simulink model "truckaso2"  (R2022b)
settings: Solver=ode3  StartTime=0.0  StopTime=Timesim  FixedStep=0.1  MaxStep=0.1  RelTol=1e-3  AbsTol=1e-6
InitFcn:
  | fismovil = readfis('movil.fis');
values from neighbouring files (symbols this model uses):
  piI = 0.5*pi    (= 1.57079632679)    [Ejercicio_llegada.m]
  xf = 75    [Ejercicio_llegada.m]
  xi = 15    [Ejercicio_llegada.m]
  yf = 75    [Ejercicio_llegada.m]
  yi = 15    [Ejercicio_llegada.m]
libraries: fuzblock x1
settings Model: Creator=pascal  LastModifiedBy=Asus_Pc
settings SolverCC: AutoScaleAbsTol=off  AlgebraicLoopSolver=TrustRegion
settings DataIOCC: SaveFormat=Array  SignalLoggingSaveFormat=ModelDataLogs  SaveOutput=off  SaveTime=off  ReturnWorkspaceOutputs=off
settings OptimizationCC: BlockReduction=off  BooleanDataType=off  ExpressionDepthLimit=2147483647  InitFltsAndDblsToZero=on  LifeSpan=inf
settings DebuggingCC: SaveWithParameterizedLinksMsg=none  UnderspecifiedInitializationDetection=Classic  MergeDetectMultiDrivingBlocksExec=none  SignalResolutionControl=TryResolveAllWithWarning  MultiTaskDSMMsg=warning  MultiTaskCondExecSysMsg=none  FcnCallInpInsideContextMsg=warning  UnconnectedInputMsg=warning  UnconnectedOutputMsg=warning  UnconnectedLineMsg=warning  StateNameClashWarn=warning  SFUnexpectedBacktrackingDiag=warning  SFNoUnconditionalDefaultTransitionDiag=warning  SFExecutionAtInitializationDiag=none  ArithmeticOperatorsInVariantConditions=warning
settings HardwareCC: ProdBitPerPointer=32  ProdBitPerSizeT=32  ProdBitPerPtrDiffT=32  ProdLargestAtomicFloat=None  ProdIntDivRoundTo=Undefined  ProdEndianess=Unspecified  ProdWordSize=32  ProdHWDeviceType=32-bit Generic  TargetUnknown=on
settings ModelReferenceCC: PropagateSignalLabelsOutOfModel=off
settings SFSimCC: SimUseLocalCustomCode=off  CustomCodeUndefinedFunction=UseInterfaceOnly
settings RTWCC: TemplateMakefile=grt_vc.tmf  RTWUseLocalCustomCode=off
settings CodeAppCC: StateflowObjectComments=on
settings GRTTargetCC: TargetFcnLib=ansi_tfl_tmw.mat  TargetLangStandard=C89/C90 (ANSI)  CombineOutputUpdateFcns=off  GRTInterface=on
settings ConfigComp: CovMetricSettings=dw  CovSaveCumulativeToWorkspaceVar=on  CovSaveSingleToWorkspaceVar=on  CovExternalEMLEnable=off

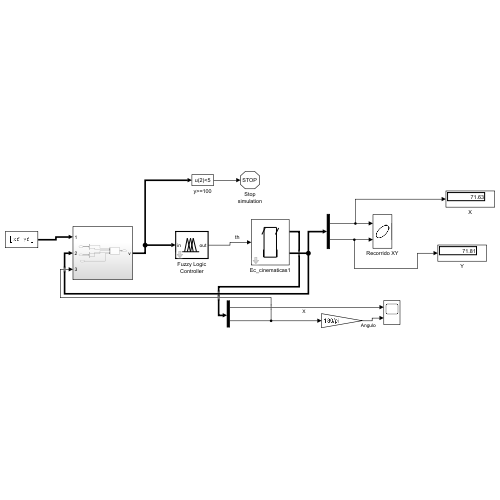
[thumbnail: Simulink's stored preview of the top-level diagram]
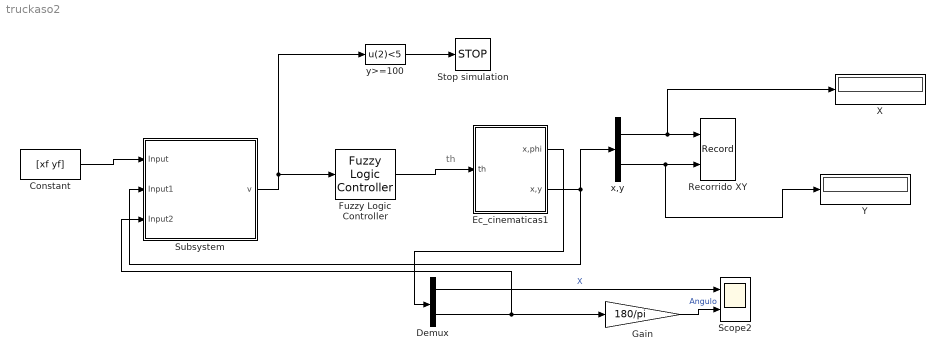
== system truckaso2 ==
  note: th
  Constant : Constant  Value=[xf yf]
  Demux : Demux  Outputs=2
  Ec_cinematicas1 : Subsystem  mask{X=xi, Y=yi, Phi=piI, D=2}
      mask prompts: X "Posición inicial X (0-100 cm):"; Y "Posición inical Y (0-100 cm):"; Phi "Orientación inicial Phi (-pi/2 a 3pi/2):"; D "Desplazamiento"
      mask Display: plot(-3, -3, 3, 3,[-1 1 1 -1 -1],[-2 -2 2 2 -2],[-1.1 -1.1],[-2 -1],[1.1 1.1],[-2 -1],[1.35 0.85],[1.93 1.07],[-0.85 -1.35],[1.93 1.07])
  Fuzzy Logic Controller : fuzblock/Fuzzy Logic  Controller  FIS=fismovil3  OutputSampleNumber=101  DataType=double  FuzzifiedInputs=off  RuleFiringStrengths=off  RuleOutputs=off  AggregatedOutputs=off  SimulateUsing=Interpreted execution  OutOfRangeInputValueMessage=warning  NoRuleFiredMessage=warning  EmptyOutputFuzzySetMessage=warning
  Gain : Gain  Gain=180/pi
  Recorrido XY : Record  FileSettingsInternal="{\"entries\":[{\"content\":{\"excelSettings\":{\"content\":{},\"type\":\"Streamout.ExcelSettings\"}},\"type\":\"Streamout.FileSettingStorage\",\"uuid\":\"7dcdacd9-9091-49d9-9ea7-95d86a0943a3\"}],\"packageUris\":[\"http://schema.mathworks.com/mf0/streamout_blocks/R2020a\"],\"version\":\"1.0\"}"  Layout=[1 1]  SignalsInternal="{\"entries\":[{\"content\":{\"signals\":[{\"content\":{\"blockPath\":[\"truckaso2/Recorrido XY\"],\"channel\":[],\"dimensions\":[1],\"domain\":\"truckaso2/Recorrido XY\",\"lineColor\":\"#a2142f\",\"plots\":[1],\"port\":1,\"sid\":[\"\"],\"signalID\":39,\"signalName\":\"x,y:1\"},\"type\":\"RecordBlkView.Signal\",\"uuid\":\"6f5dfcf6-7128-426f-a57b-a5e084615930\"},{\"content\":{\"blockPath\":[\"truckaso2/Recorrido XY\"],\"channel\":[],\"dimensions\":[1],\"domain\":\"truckaso2/Recorrido XY\",\"lineColor\":\"#139fff\",\"plots\":[1],\"port\":2,\"sid\":[\"\"],\"signalID\":43,\"signalName\":\"x,y:2\"},\"type\":\"RecordBlkView.Signal\",\"uuid\":\"7ab47a85-be80-48e0-8b0c-3861602a2193\"}]},\"type\":\"RecordBlkView.InputSignals\",\"uuid\":\"6bd8f785-4fa3-407f-9c70-a3b5344d18c7\"}],\"packageUris\":[\"http://schema.mathworks.com/mf0/streamout_blocks/R2020a\"],\"version\":\"1.0\"}"  VisualizationBindings="{\"xyplotplugin\":{\"info\":[{\"series\":[{\"bindingParametersList\":[{\"parameter\":\"X-Axis\",\"signalID\":39,\"signalName\":\"x,y:1\"},{\"parameter\":\"Y-Axis\",\"signalID\":43,\"signalName\":\"x,y:2\"}],\"seriesID\":36838}],\"subplotID\":1}]}}"  CompatibilityTag=XY  st=-1
  Scope2 : Scope  NumInputPorts=2
  Stop simulation : Stop
  Subsystem : Subsystem
  X : Display
  Y : Display
  x,y : Demux  Outputs=2
  y>=100 : Fcn  Expr=u(2)<5
  wires:
  x,y/2 -> Y/1, Recorrido XY/2
  Fuzzy Logic Controller/1 -> Ec_cinematicas1/1(th)
  x,y/1 -> X/1, Recorrido XY/1
  Constant/1 -> Subsystem/1(Input)
  Subsystem/1(v) -> y>=100/1, Fuzzy Logic Controller/1
  y>=100/1 -> Stop simulation/1
  Demux/2 -> Subsystem/3(Input2), Gain/1
  Demux/1 -> Scope2/1  "X"
  Gain/1 -> Scope2/2  "Angulo"
  Ec_cinematicas1/1(x,phi) -> Demux/1
  Ec_cinematicas1/2(x,y) -> x,y/1, Subsystem/2(Input1)

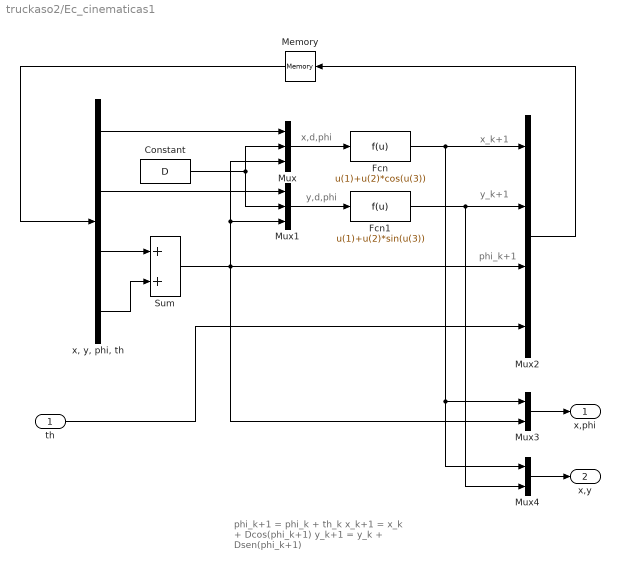
== system truckaso2/Ec_cinematicas1 ==
  note: x,d,phi
  note: x_k+1
  note: y,d,phi
  note: y_k+1
  note: phi_k+1 = phi_k + th_k
      |
      | x_k+1 = x_k + Dcos(phi_k+1)
      |
      | y_k+1 = y_k + Dsen(phi_k+1)
  note: phi_k+1
  th : Inport
  Constant : Constant  Value=D
  Fcn : Fcn  Expr=u(1)+u(2)*cos(u(3))
  Fcn1 : Fcn  Expr=u(1)+u(2)*sin(u(3))
  Memory : Memory  InitialCondition=[X Y Phi 0]
  Mux : Mux  Inputs=3
  Mux1 : Mux  Inputs=3
  Mux2 : Mux
  Mux3 : Mux  Inputs=2
  Mux4 : Mux  Inputs=2
  Sum : Sum
  "x, y, phi, th" : Demux
  x,phi : Outport
  x,y : Outport  Port=2
  wires:
  Mux/1 -> Fcn/1
  Mux1/1 -> Fcn1/1
  Fcn/1 -> Mux2/1, Mux3/1, Mux4/1
  Fcn1/1 -> Mux2/2, Mux4/2
  "x, y, phi, th"/1 -> Mux/1
  "x, y, phi, th"/2 -> Mux1/1
  "x, y, phi, th"/3 -> Sum/1
  Sum/1 -> Mux1/3, Mux/3, Mux3/2, Mux2/3
  Constant/1 -> Mux/2, Mux1/2
  Mux3/1 -> x,phi/1
  Mux4/1 -> x,y/1
  th/1 -> Mux2/4
  "x, y, phi, th"/4 -> Sum/2
  Memory/1 -> "x, y, phi, th"/1
  Mux2/1 -> Memory/1

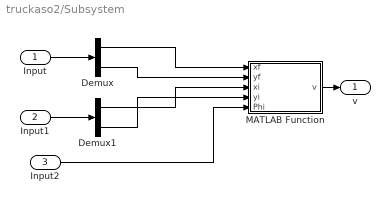
== system truckaso2/Subsystem ==
  Input : Inport
  Input1 : Inport  Port=2
  Input2 : Inport  Port=3
  Demux : Demux  Outputs=2
  Demux1 : Demux  Outputs=2
  MATLAB Function : MATLAB Function  TreatAsAtomicUnit=on
  v : Outport
  wires:
  Demux/1 -> MATLAB Function/1(xf)
  MATLAB Function/1(v) -> v/1
  Demux/2 -> MATLAB Function/2(yf)
  Input/1 -> Demux/1
  Demux1/1 -> MATLAB Function/3(xi)
  Demux1/2 -> MATLAB Function/4(yi)
  Input1/1 -> Demux1/1
  Input2/1 -> MATLAB Function/5(Phi)

== matlab function truckaso2/Subsystem/MATLAB Function ==
  data: xf input; v output; yf input; xi input; yi input; Phi input
%  Cálculo de la DISTANCIA  que separa al móvil de su
%  punto final y del ángulo GAMA necesario para calcular
%  el ángulo ALFA, perteneciente al sistema de conducción de un móvil
% u = [ xf ; yf ; xi ; yi ; Phi]
% v = [ Alfa ; Distancia ] 


function v = Dist_Gama(xf, yf, xi, yi, Phi)

% Cálculo de la distancia
  dX        = abs(xf - xi);
  dY        = abs(yf - yi); 
  distancia = sqrt(dX^2 + dY^2);
  cateto_opuesto = 0;
  Angulo_cuadrante = 0;
% Cálculo del cuadrante de operacion
  if (yf >= yi && xf > xi)
      Angulo_cuadrante = 0 ;
      cateto_opuesto   = dY ;
  end
  if (yf >= yi && xf <= xi)
      Angulo_cuadrante = pi/2 ;
      cateto_opuesto   = dX ;
  end
  if (yf < yi  && xf <= xi)
      Angulo_cuadrante = pi ;
      cateto_opuesto   = dY ;
  end
  if (yf < yi  && xf > xi)
      Angulo_cuadrante = 3*pi/2 ;
      cateto_opuesto   = dX ;
  end

% Cálculo del ángulo beta
  Beta      = asin(cateto_opuesto/distancia);
  
% Cálculo del ángulo gama
  Gama      = Beta + Angulo_cuadrante;

% Cálculo de Alfa conservando el rango entre -180 0 180
  Alfa      = Phi - Gama; 
  if  (Alfa > pi)
      Alfa  = Alfa - 2*pi;
  end
  if (Alfa < -pi)
      Alfa  = 2*pi + Alfa;
  end

  v = [Alfa;distancia];
end
